simulink model "PCG_Eval_P6_sf"  (Simulink 6.5)
settings: Solver=FixedStepDiscrete  SolverMode=SingleTasking  StartTime=0.0  StopTime=2  FixedStep=.001  MaxStep=10  RelTol=1e-3
PostLoadFcn:
  | if (exist('PCG_Demo_5_data','file'))
  |    load PCG_Demo_5_data;
  | else
  |    % Load Data Objects
  |    PCG_Eval_Base_Data_Stage_5;
  | end
CloseFcn:
  | rtwprivate ssgencode ModelCloseRequest PCG_Eval_P1
settings Model: Creator=mburke  LastModifiedBy=mburke  ProdHWDeviceType=32-bit Embedded Processor
settings DataIOCC: LimitDataPoints=off  SaveFormat=StructureWithTime  SaveOutput=off  SaveTime=off
settings OptimizationCC: InlineParams=on  LifeSpan=1
settings DebuggingCC: CheckExecutionContextPreStartOutputMsg=on  CheckExecutionContextRuntimeOutputMsg=on  SignalResolutionControl=UseLocalSettings  IntegerOverflowMsg=none  InvalidFcnCallConnMsg=warning  StrictBusMsg=ErrorLevel1
settings HardwareCC: ProdHWDeviceType=32-bit Embedded Processor
settings ModelReferenceCC: ModelReferenceNumInstancesAllowed=Single  ModelReferencePassRootInputsByReference=off

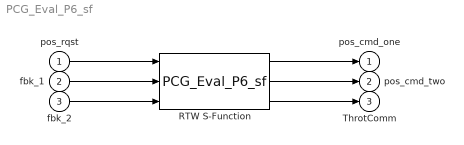
== system PCG_Eval_P6_sf ==
  note: Copyright 2007 The MathWorks, Inc.
  note: Copyright 2007 The MathWorks, Inc.
  pos_rqst : Inport
  fbk_1 : Inport  Port=2
  fbk_2 : Inport  Port=3
  RTW S-Function : S-Function  FunctionName=PCG_Eval_P6_sf  SFunctionModules=""  mask{rtw_sf_name=PCG_Eval_P6_sf, showVar=off}
      mask prompts: rtw_sf_name "Generated S-function name (model_sf):"; showVar "Show module list"
      mask help: Real-Time Workshop generated S-function.
      mask init:
      | displist = '';
      | if ~strcmp(get_param(gcb, 'FunctionName'), rtw_sf_name);
      |   set_param(gcb, 'FunctionName', rtw_sf_name);
      | end
      | % Check if we are generating RTW code
      | rtw_mode = false;
      | if strcmpi(get_param(bdroot(gcb),'SimulationStatus'),'Initializing')
      | 	rtw_mode = strcmpi(get_param(bdroot(gcb),'BuildingRTWCode'),'on') && ...
      | 		~strcmpi(get_param(bdroot(gcb),'TargetStyle'),'SimulationTarget');
      | end
      | if showVar || rtw_mode
      | 	if exist('rtwsfunc') == 2 | exist('rtwsfunc') == 6
      | 		tmplist = rtwsfunc(rtw_sf_name,gcb);
      | 		tmplist = ['\nList of Modules:\n', tmplist];
      | 	elseif showVar
      | 		tmplist = '\nList of Modules:\nRTW not licensed\n';
      |  	end
      | end
      | if showVar
      |   displist = tmplist;
      | end
      settings: CopyFcn=set_param(gcb,'LinkStatus','none');
      mask Help: helpview([docroot,'\toolbox\rtw\helptargets.map'],'rtw_Sfunc_target');
      mask Display:
      | port_label('input',1,'pos_rqst');
      | port_label('input',2,'fbk_1');
      | port_label('input',3,'fbk_2');
      | port_label('output',1,'pos_cmd_one');
      | port_label('output',2,'pos_cmd_two');
      | port_label('output',3,'ThrotComm');
  pos_cmd_one : Outport
  pos_cmd_two : Outport  Port=2
  ThrotComm : Outport  Port=3  UseBusObject=on  BusOutputAsStruct=on
      settings: BusObject=ThrottleCommands
  wires:
  pos_rqst/1 -> RTW S-Function/1
  fbk_1/1 -> RTW S-Function/2
  fbk_2/1 -> RTW S-Function/3
  RTW S-Function/1 -> pos_cmd_one/1
  RTW S-Function/2 -> pos_cmd_two/1
  RTW S-Function/3 -> ThrotComm/1
